simulink model "modelo"  (R2020b)
settings: Solver=VariableStepAuto  StartTime=0.0  StopTime=60.0  RelTol=1e-3
undefined symbols (not defined in the file): sigbuilder_block
settings Model: Creator=dougl  LastModifiedBy=dougl

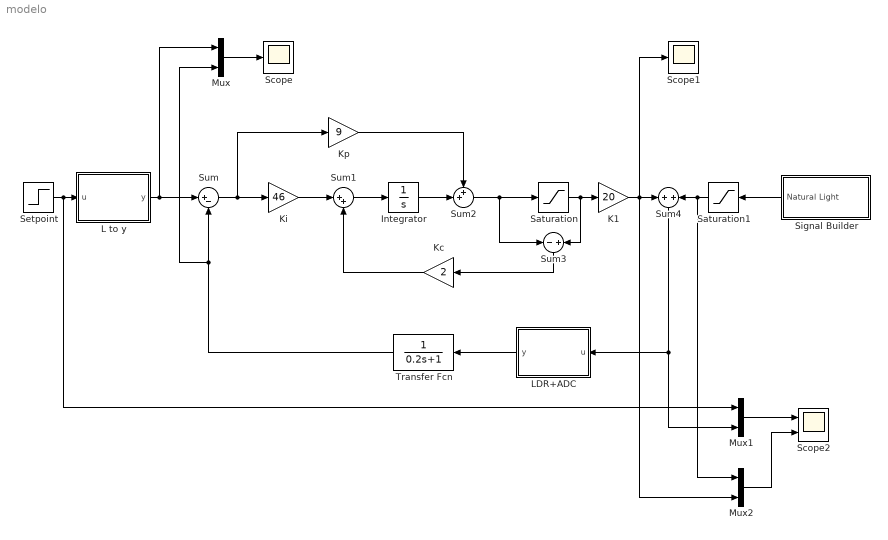
== system modelo ==
  Integrator : Integrator
  K1 : Gain  Gain=20
  Kc : Gain  Gain=2
  Ki : Gain  Gain=46
  Kp : Gain  Gain=9
  L to y : MATLAB Function  TreatAsAtomicUnit=on
  LDR+ADC : MATLAB Function  TreatAsAtomicUnit=on
  Mux : Mux  Inputs=2
  Mux1 : Mux  Inputs=2
  Mux2 : Mux  Inputs=2
  Saturation : Saturate
  Saturation1 : Saturate  UpperLimit=1100
  Scope : Scope
  Scope1 : Scope
  Scope2 : Scope  NumInputPorts=2
  Setpoint : Step  Time=20  Before=300  After=800  SampleTime=0
  Signal Builder : Subsystem  Tag=STV Subsys  LoadFcn=sigbuilder_block('load');  StartFcn=sigbuilder_block('start');  StopFcn=sigbuilder_block('stop');  ClipboardFcn=sigbuilder_block('clipboard');  mask(Sigbuilder block){tuvar=[0:10]}
      mask help: Simulink:masks:SigbuilderBlock_MD
      mask init:
      | if ~strcmp(get_param(bdroot(gcbh),'SimulationStatus'),'stopped') tuvar = sigbuilder_block('maskInit'); end
      settings: CopyFcn=sigbuilder_block('copy');  DeleteFcn=sigbuilder_block('delete');  ModelCloseFcn=sigbuilder_block('modelClose');  PreSaveFcn=sigbuilder_block('preSave');  PauseFcn=sigbuilder_block('pause');  ContinueFcn=sigbuilder_block('continue');  NameChangeFcn=sigbuilder_block('namechange');  OpenFcn=sigbuilder_block('open',[144.75 216.75 528.75 399.75 ]);  CloseFcn=sigbuilder_block('close');
      mask Display: plot(0, 0, 100, 100,[2, 2, 32, 32, 2], [68, 8, 8, 68, 68],[32, 2], [38, 38], [32, 19, 2],[53, 60, 44], [32, 17, 17, 2],[16, 16, 31, 31]);txt = getActiveGroup(gcbh);text(2, 100, txt,'verticalAlignment', 'top');
  Sum : Sum  Inputs=|+-
  Sum1 : Sum  Inputs=|++
  Sum2 : Sum  Inputs=++|
  Sum3 : Sum  Inputs=-|+
  Sum4 : Sum  Inputs=+|+
  Transfer Fcn : TransferFcn  Denominator=[0.2 1]
  wires:
  Mux/1 -> Scope/1
  Setpoint/1 -> Mux1/1, L to y/1(u)
  L to y/1(y) -> Mux/1, Sum/1
  Sum/1 -> Kp/1, Ki/1
  Ki/1 -> Sum1/1
  Sum1/1 -> Integrator/1
  Kc/1 -> Sum1/2
  Integrator/1 -> Sum2/2
  Kp/1 -> Sum2/1
  Sum2/1 -> Sum3/1, Saturation/1
  Sum3/1 -> Kc/1
  Saturation/1 -> Sum3/2, K1/1
  K1/1 -> Mux2/2, Scope1/1, Sum4/1
  Saturation1/1 -> Mux2/1, Sum4/2
  Sum4/1 -> Mux1/2, LDR+ADC/1(u)
  LDR+ADC/1(y) -> Transfer Fcn/1
  Transfer Fcn/1 -> Mux/2, Sum/2
  Signal Builder/1(Natural Light) -> Saturation1/1
  Mux1/1 -> Scope2/1
  Mux2/1 -> Scope2/2

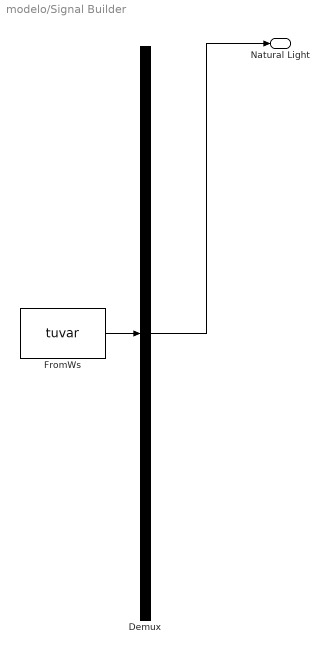
== system modelo/Signal Builder ==
  Demux : Demux  Tag=STV Demux  Outputs=1
      settings: DisplayOption=none
  FromWs : FromWorkspace  Tag=STV FromWs  VariableName=tuvar
      SigBuilderData=|
      | common.afterFinalStr = 'Extrapolate'
      | common.sampleTime = 0
      | dataSet.timeRange = [0 60]
      | dataSet.name = 'Group 1'
      | sbobj.Groups.Name = 'Group 1'
      | sbobj.Groups.Signals.Name = 'Natural Light'
      | sbobj.Groups.Signals.XData = [0 10 10 25 25 40 40 50 50 60]
      | sbobj.Groups.Signals.YData = [11 11 400 400 1003.02 1000 200 200 11 11]
      | sbobj.Groups.TimeRange = [0 60]
  Natural Light : Outport  Tag=STV Outport
  wires:
  Demux/1 -> Natural Light/1
  FromWs/1 -> Demux/1

== matlab function modelo/L to y ==
  data: u input; y output
function y = fcn(u)
y = 0.3443*log(u)-0.158;

== matlab function modelo/LDR+ADC ==
  data: u input; y output
function y = fcn(u)
R1 = 400;
R2 = 9e3;
L1 = 1000;
L2 = 10;
R0 = 2.2e3;

k = (log(R1)-log(R2))/(log(L1)-log(L2));
m = (log(R2)*log(L1)-log(R1)*log(R2))/(log(L1)-log(L2));
y = R0/(R0+10^(k*log(u)+m));
